simulink model "sensor_2"  (R2018a)
settings: Solver=FixedStepAuto  StartTime=0.0  StopTime=time_end  FixedStep=dt  RelTol=1e-3
values from neighbouring files (symbols this model uses):
  tau = 1/(2*pi*0.2)    (= 0.795774715459)    [sim_sensor.m]    (also in sim_sensor_2.m)
settings Model: Creator=aoki-soya  LastModifiedBy=aoki-soya

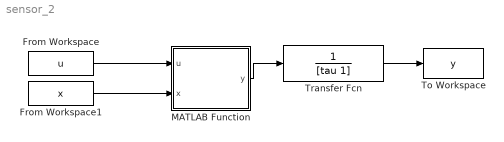
== system sensor_2 ==
  From Workspace : FromWorkspace  VariableName=u  SampleTime=0
  From Workspace1 : FromWorkspace  VariableName=x  SampleTime=0
  MATLAB Function : MATLAB Function  TreatAsAtomicUnit=on
  To Workspace : ToWorkspace  VariableName=y  SaveFormat=Timeseries  SampleTime=-1
  Transfer Fcn : TransferFcn  Denominator=[tau 1]
  wires:
  From Workspace/1 -> MATLAB Function/1(u)
  From Workspace1/1 -> MATLAB Function/2(x)
  MATLAB Function/1(y) -> Transfer Fcn/1
  Transfer Fcn/1 -> To Workspace/1

== matlab function sensor_2/MATLAB Function ==
  settings: updateMethod=DISCRETE  sampleTime=dt
  data: u input; y output; x input
function y = sensor(u,x)

% mu & sigma
GPR_mu = loadCompactModel('GPR_mu');
GPR_sigma = loadCompactModel('GPR_sigma');
[mu_pred,~,mu_int] = predict(GPR_mu,[x,1]);
[sigma_pred,~,sigma_int] = predict(GPR_sigma,[x,1]);

y = normrnd(sign(u)*(abs(u)+mu_pred), sigma_pred);
